simulink model "rc_blink_sim2"  (R2017a)
settings: Solver=FixedStepAuto  StartTime=0.0  StopTime=30.0  RelTol=1e-3  EnableMultiTasking=on
libraries: simulink x1
settings Model: Creator=Parker  LastModifiedBy=Parker
settings SolverCC: PositivePriorityOrder=on
settings OptimizationCC: PassReuseOutputArgsAs=Individual arguments  MaxStackSize=64
settings DebuggingCC: ParameterTunabilityLossMsg=error
settings HardwareCC: ProdBitPerPointer=32  ProdBitPerSizeT=32  ProdBitPerPtrDiffT=32  ProdLargestAtomicInteger=Long  ProdLargestAtomicFloat=Double  ProdWordSize=32  ProdHWDeviceType=ARM Compatible->ARM Cortex
settings SFSimCC: MATLABDynamicMemAlloc=off
settings RTWCC: SystemTargetFile=ert.tlc  HardwareBoard=Raspberry Pi  TLCOptions="-aInlineSetEventsForThisBaseRateFcn=TLC_FALSE -aSuppressMultiTaskScheduler=TLC_FALSE  -aRateBasedStepFcn=0"  TemplateMakefile=ert_default_tmf  Description=Embedded Coder  GenerateReport=on  Toolchain=GNU GCC Raspberry Pi  IncludeHyperlinkInReport=on  LaunchReport=on  GenerateTraceInfo=on  GenerateTraceReport=on  GenerateTraceReportSl=on  GenerateTraceReportSf=on  GenerateTraceReportEml=on
settings CodeAppCC: ForceParamTrailComments=on  IgnoreCustomStorageClasses=off  OperatorAnnotations=on  SimulinkDataObjDesc=on  SFDataObjDesc=on  MATLABFcnDesc=on  InsertBlockDesc=on  MATLABSourceComments=on
settings ERTTargetCC: SupportVariableSizeSignals=on

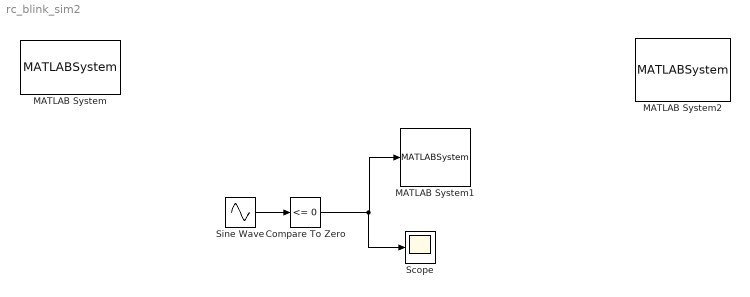
== system rc_blink_sim2 ==
  Compare To Zero : simulink/Logic and Bit Operations/Compare To Zero  relop=<=  OutDataTypeStr=uint8
  MATLAB System : MATLABSystem  System=rc_initialize_sys
      mask Type: rc_initialize_sys
      mask Display: disp('rc_initialize_sys');
  MATLAB System1 : MATLABSystem  System=rc_set_led  rc_led_t=1
      mask Type: rc_set_led
      mask Display:
      | disp('rc_set_led');
      | port_label('input',1,'u');
  MATLAB System2 : MATLABSystem  System=rc_cleanup_sys
      mask Type: rc_cleanup_sys
      mask Display: disp('rc_cleanup_sys');
  Scope : Scope
  Sine Wave : Sin  SineType=Sample based  Amplitude=20  Frequency=2  Samples=20  SampleTime=0.1
  wires:
  Sine Wave/1 -> Compare To Zero/1
  Compare To Zero/1 -> Scope/1, MATLAB System1/1
